simulink model "L4_4"  (R2023a)
settings: Solver=VariableStepAuto  StartTime=0.0  StopTime=100  RelTol=1e-8
undefined symbols (not defined in the file): k
settings Model: Creator=apere  LastModifiedBy=apere

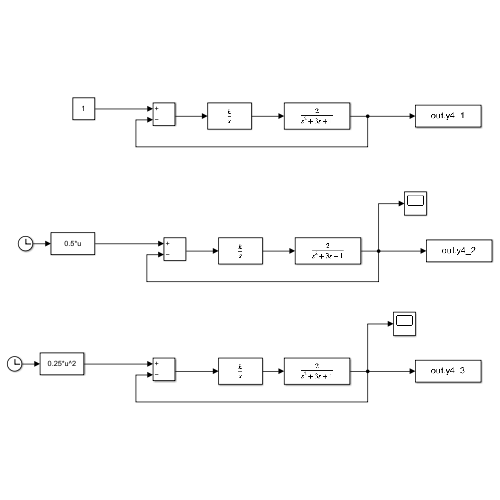
[thumbnail: Simulink's stored preview of the top-level diagram]
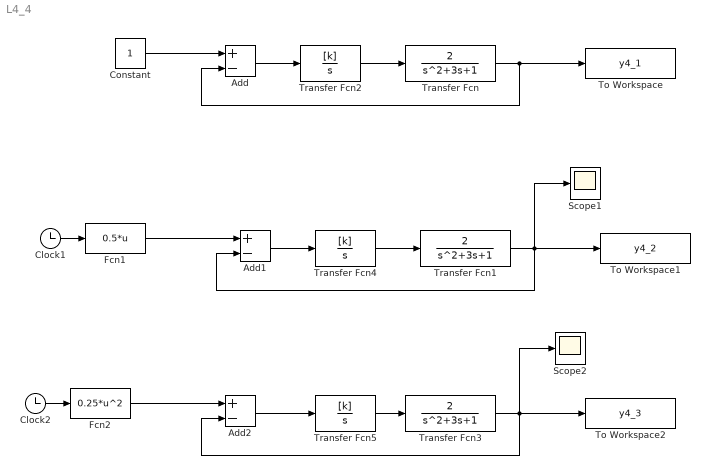
== system L4_4 ==
  Add : Sum  Inputs=+-
  Add1 : Sum  Inputs=+-
  Add2 : Sum  Inputs=+-
  Clock1 : Clock
  Clock2 : Clock
  Constant : Constant
  Fcn1 : Fcn  Expr=0.5*u
  Fcn2 : Fcn  Expr=0.25*u^2
  Scope1 : Scope
  Scope2 : Scope
  To Workspace : ToWorkspace  VariableName=y4_1  SaveFormat=Timeseries  SampleTime=-1
  To Workspace1 : ToWorkspace  VariableName=y4_2  SaveFormat=Timeseries  SampleTime=-1
  To Workspace2 : ToWorkspace  VariableName=y4_3  SaveFormat=Timeseries  SampleTime=-1
  Transfer Fcn : TransferFcn  Numerator=[2]  Denominator=[1 3 1]
  Transfer Fcn1 : TransferFcn  Numerator=[2]  Denominator=[1 3 1]
  Transfer Fcn2 : TransferFcn  Numerator=[k]  Denominator=[1 0]
  Transfer Fcn3 : TransferFcn  Numerator=[2]  Denominator=[1 3 1]
  Transfer Fcn4 : TransferFcn  Numerator=[k]  Denominator=[1 0]
  Transfer Fcn5 : TransferFcn  Numerator=[k]  Denominator=[1 0]
  wires:
  Constant/1 -> Add/1
  Transfer Fcn/1 -> To Workspace/1, Add/2
  Fcn1/1 -> Add1/1
  Add/1 -> Transfer Fcn2/1
  Transfer Fcn4/1 -> Transfer Fcn1/1
  Add1/1 -> Transfer Fcn4/1
  Clock1/1 -> Fcn1/1
  Transfer Fcn2/1 -> Transfer Fcn/1
  Transfer Fcn1/1 -> To Workspace1/1, Add1/2, Scope1/1
  Transfer Fcn3/1 -> To Workspace2/1, Add2/2, Scope2/1
  Fcn2/1 -> Add2/1
  Clock2/1 -> Fcn2/1
  Add2/1 -> Transfer Fcn5/1
  Transfer Fcn5/1 -> Transfer Fcn3/1
